simulink model "PROVA_IMU"  (R2023b)
settings: Solver=ode1  StartTime=0.0  StopTime=inf  FixedStep=.004  RelTol=1e-3  EnableMultiTasking=on
values from neighbouring files (symbols this model uses):
  soglia_nonlin = 0.5    [model_params.m]
undefined symbols (not defined in the file or in its folder): deg, m, s
libraries: CP_library x1, QB_pacer_lib x1, qbmove_library x1, vrlib x1
settings Model: Creator=laurentio  LastModifiedBy=ilari
settings SolverCC: AlgebraicLoopSolver=TrustRegion
settings DataIOCC: LimitDataPoints=on  SaveFormat=Array  ReturnWorkspaceOutputs=off
settings OptimizationCC: LifeSpan=inf
settings DebuggingCC: UnderspecifiedInitializationDetection=Classic  MergeDetectMultiDrivingBlocksExec=none  SolverPrmCheckMsg=warning  UnconnectedInputMsg=warning  UnconnectedOutputMsg=warning  UnconnectedLineMsg=warning  AllowSymbolicDim=off  StateNameClashWarn=warning  SFUnexpectedBacktrackingDiag=warning  SFNoUnconditionalDefaultTransitionDiag=warning  SFExecutionAtInitializationDiag=none  ArithmeticOperatorsInVariantConditions=warning
settings HardwareCC: ProdBitPerPointer=32  ProdBitPerSizeT=32  ProdBitPerPtrDiffT=32  ProdLargestAtomicFloat=None  ProdIntDivRoundTo=Undefined  ProdEndianess=Unspecified  ProdWordSize=32  ProdHWDeviceType=32-bit Generic
settings ModelReferenceCC: EnableRefExpFcnMdlSchedulingChecks=on  PropagateSignalLabelsOutOfModel=off
settings SFSimCC: SimUseLocalCustomCode=off  CustomCodeUndefinedFunction=UseInterfaceOnly
settings RTWCC: RTWUseLocalCustomCode=off  DLArmComputeVersion=19.05
settings CodeAppCC: StateflowObjectComments=on
settings GRTTargetCC: TargetLangStandard=C89/C90 (ANSI)
settings ConfigComp: CovMetricSettings=dw  CovSaveCumulativeToWorkspaceVar=on  CovSaveSingleToWorkspaceVar=on  CovExternalEMLEnable=off  CovSFcnEnable=off

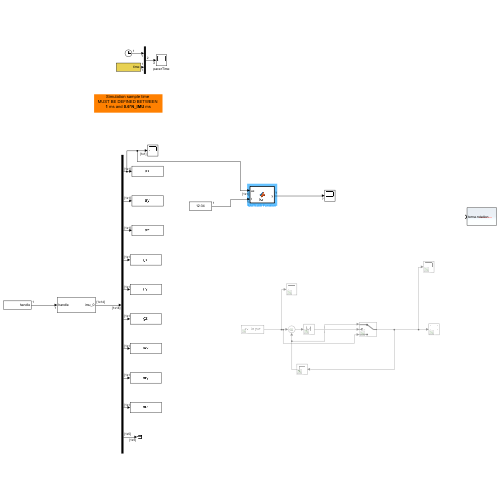
[thumbnail: Simulink's stored preview of the top-level diagram]
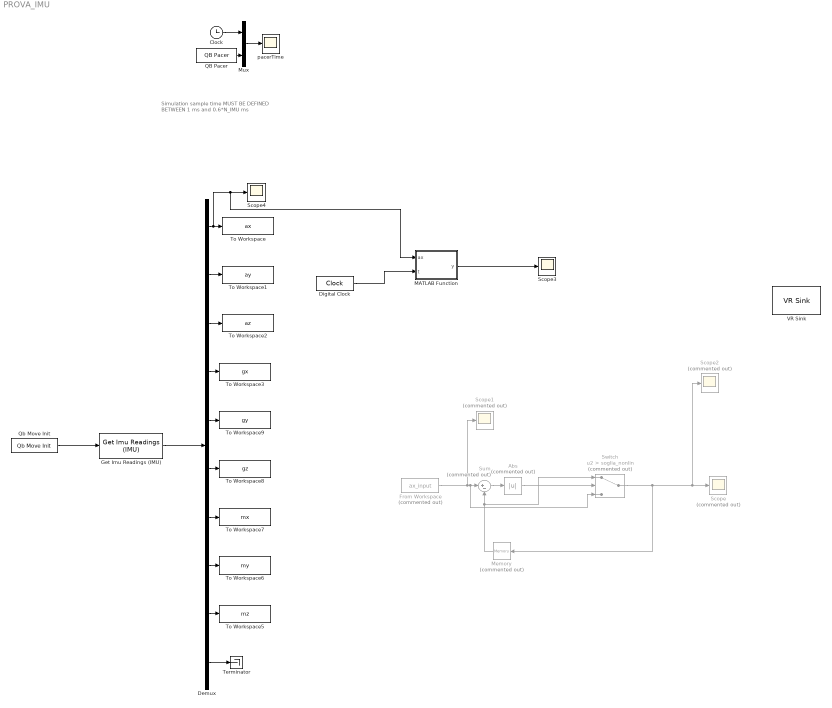
== system PROVA_IMU ==
  note: Simulation sample time
      | MUST BE DEFINED BETWEEN
      | 1 ms and 0.6*N_IMU ms
  Abs : Abs  Commented=on  SaturateOnIntegerOverflow=off
  Clock : Clock
  Demux : Demux  Outputs=[1 1 1 1 1 1 1 1 1 5 ]
  Digital Clock : DigitalClock
  From Workspace : FromWorkspace  Commented=on  VariableName=ax_input
  Get Imu Readings (IMU) : CP_library/Get Imu Readings (IMU)  ID=2  N_IMU=1  DAISY_CHAINING=off  ACC_UNITY=m/(s^2)  GYRO_UNITY=deg/s  MAG_UNITY=uT
      settings: SourceProductName=Centro Piaggio Library
  MATLAB Function : MATLAB Function  TreatAsAtomicUnit=on
  Memory : Memory  Commented=on  InitialCondition=7
  Mux : Mux  Inputs=2
  QB Pacer : QB_pacer_lib/QB Pacer  simTimePerRealTime=1
      settings: SourceProductName=QB Pacer
  Qb Move Init : qbmove_library/Qb Move Init  NUMBER_OF_COM='COM9'  BAUD_RATE_COM=2000000
      settings: SourceProductName=Qb Move Library
  Scope : Scope  Commented=on
  Scope1 : Scope  Commented=on
  Scope2 : Scope  Commented=on
  Scope3 : Scope
  Scope4 : Scope
  Sum : Sum  Commented=on  Inputs=|+-
  Switch : Switch  Commented=on  Criteria=u2 > Threshold  Threshold=soglia_nonlin  SaturateOnIntegerOverflow=off  InputSameDT=off
  Terminator : Terminator
  To Workspace : ToWorkspace  VariableName=ax  SaveFormat=Timeseries  SampleTime=-1
  To Workspace1 : ToWorkspace  VariableName=ay  SaveFormat=Timeseries  SampleTime=-1
  To Workspace2 : ToWorkspace  VariableName=az  SaveFormat=Timeseries  SampleTime=-1
  To Workspace3 : ToWorkspace  VariableName=gx  SaveFormat=Timeseries  SampleTime=-1
  To Workspace5 : ToWorkspace  VariableName=mz  SaveFormat=Timeseries  SampleTime=-1
  To Workspace6 : ToWorkspace  VariableName=my  SaveFormat=Timeseries  SampleTime=-1
  To Workspace7 : ToWorkspace  VariableName=mx  SaveFormat=Timeseries  SampleTime=-1
  To Workspace8 : ToWorkspace  VariableName=gz  SaveFormat=Timeseries  SampleTime=-1
  To Workspace9 : ToWorkspace  VariableName=gy  SaveFormat=Timeseries  SampleTime=-1
  VR Sink : vrlib/VR Sink  InstantiateOnLoad=on  SampleTime=0.1  ViewEnable=on  RemoteChange=off  RemoteView=off  FieldsWritten=terna.rotation.4.1.1.double  WorldFileName=irene.wrl  AutoView=off  VideoDimensions=[]  AllowVariableSize=off
  pacerTime : Scope
  wires:
  QB Pacer/1 -> Mux/2
  Clock/1 -> Mux/1
  Qb Move Init/1 -> Get Imu Readings (IMU)/1
  Mux/1 -> pacerTime/1
  Get Imu Readings (IMU)/1 -> Demux/1
  Demux/3 -> To Workspace2/1
  Demux/2 -> To Workspace1/1
  Demux/1 -> To Workspace/1, MATLAB Function/1(ax), Scope4/1
  Demux/4 -> To Workspace3/1
  Demux/5 -> To Workspace9/1
  Demux/6 -> To Workspace8/1
  Demux/7 -> To Workspace7/1
  Demux/8 -> To Workspace6/1
  Demux/9 -> To Workspace5/1
  Demux/10 -> Terminator/1
  Switch/1 -> Memory/1, Scope2/1, Scope/1
  From Workspace/1 -> Scope1/1, Switch/3, Sum/1
  Memory/1 -> Sum/2, Switch/1
  Sum/1 -> Abs/1
  Abs/1 -> Switch/2
  MATLAB Function/1(y) -> Scope3/1
  Digital Clock/1 -> MATLAB Function/2(t)

== matlab function PROVA_IMU/MATLAB Function ==
  data: ax input; y output; t input
function y = fcn(ax , t)

if cont == 0;
    ax_pre = ax;
end

if abs(ax-ax_pre)> 2
    y = ax_pre;
else 
    y = ax;

end
cont = cont+1;
ax_pre = ax;
